simulink model "cantx_4X"  (R2022b)
settings: configuration reference "SLDD_CFG" (kept outside this file)
libraries: user_lib x2, simulink x1
settings Model: DataDictionary=cantx_4X.sldd  Creator=Castiel  LastModifiedBy=Castiel
settings ConfigSetRef: SourceName=SLDD_CFG

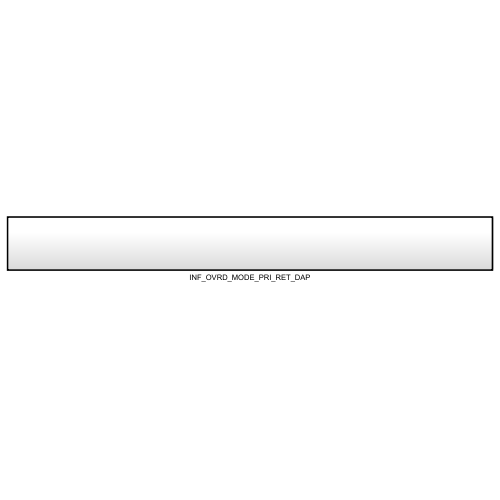
[thumbnail: Simulink's stored preview of the top-level diagram]
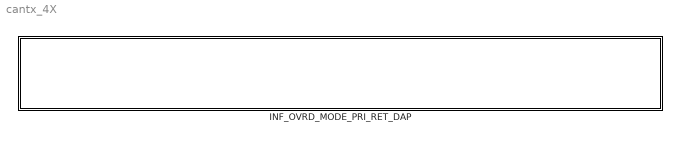
== system cantx_4X ==
  INF_OVRD_MODE_PRI_RET_DAP : Subsystem  TreatAsAtomicUnit=on
      settings: RTWSystemCode=Nonreusable function

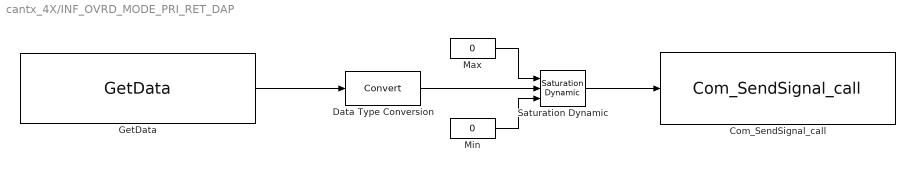
== system cantx_4X/INF_OVRD_MODE_PRI_RET_DAP ==
  Com_SendSignal_call : user_lib/Com_SendSignal_call  signalId=id2
      settings: SourceProductName=User Defined for IFLayer
  Data Type Conversion : DataTypeConversion  ConvertRealWorld=Stored Integer (SI)  SaturateOnIntegerOverflow=off  RndMeth=Floor
  GetData : user_lib/GetData  interface=INF_OVRD_MODE_PRI_RET_DAP  signalType=UB
      settings: SourceProductName=User Defined for IFLayer
  Max : Constant  Value=0  OutDataTypeStr=Inherit: Inherit via back propagation
  Min : Constant  Value=0  OutDataTypeStr=Inherit: Inherit via back propagation
  Saturation Dynamic : simulink/Discontinuities/Saturation Dynamic  OutMin=[]  OutMax=[]  OutDataTypeStr=Inherit: Same as second input  OutDataType=fixdt(1, 16)  OutScaling=2^-10  DoSatur=off
  wires:
  Saturation Dynamic/1 -> Com_SendSignal_call/1
  Min/1 -> Saturation Dynamic/3
  Max/1 -> Saturation Dynamic/1
  GetData/1 -> Data Type Conversion/1
  Data Type Conversion/1 -> Saturation Dynamic/2
